simulink model "PV_Mathematical_Model_No_Load"  (R2022a)
settings: Solver=FixedStepAuto  StartTime=0.0  StopTime=5  FixedStep=1e-5  RelTol=1e-3
libraries: simulink x1, spspowerguiLib x1
settings Model: Creator=nikos  LastModifiedBy=nikos

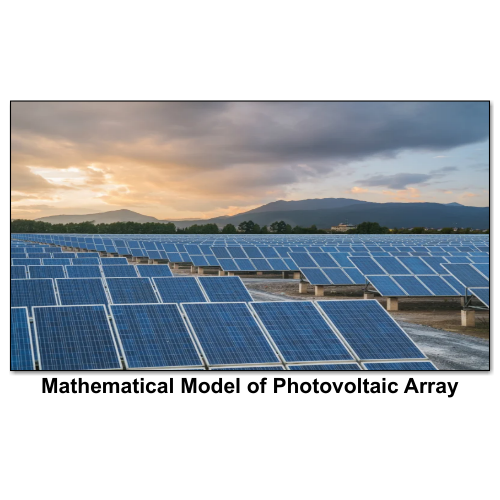
[thumbnail: Simulink's stored preview of the top-level diagram]
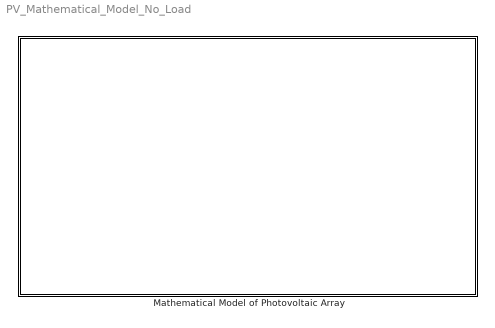
== system PV_Mathematical_Model_No_Load ==
  Mathematical Model of Photovoltaic Array : Subsystem
      mask Display: image('$imagefile'); % Use "Edit Image" on toolstrip to change.

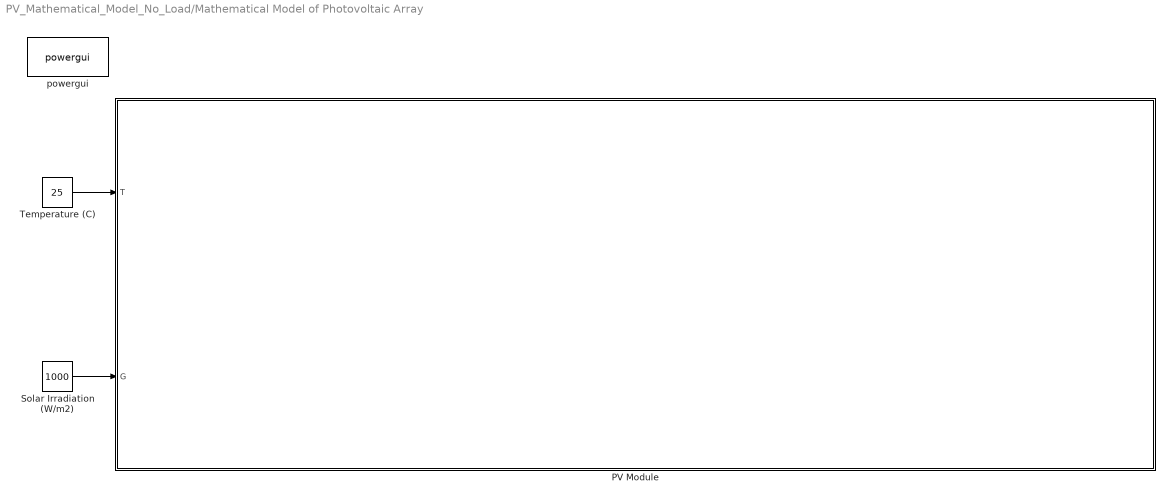
== system PV_Mathematical_Model_No_Load/Mathematical Model of Photovoltaic Array ==
  PV Module : Subsystem
  Solar Irradiation (W/m2) : Constant  Value=1000
  Temperature (C) : Constant  Value=25
  powergui : spspowerguiLib/powergui  Priority=1  SimulationMode=Discrete  SampleTime=50e-6  frequency=60  Iterations=50  frequencyindice=0  Pbase=100e6  ErrMax=1e-4  UnitsV=kV  UnitsW=MW  buscounter=0  FunctionMessages=off  echomessages=off  EnableUseOfTLC=off  CurrentSourceSwitches=off  DisableSnubberDevices=off  DisableRonSwitches=off  DisableVfSwitches=off  DisplayEquations=off  AutomaticDiscreteSolvers=off  SolverType=Tustin/Backward Euler (TBE)  Interpol=off  ExternalGateDelay=off  methode=off  Ts=100  x0status=blocks  SPID=on  SwTol=0  HookPort=off  NonlinearTolerance=1e-4  nMaxIteration=100  ContinueOnMaxIteration=off  RestoreLinks=warning  ResistiveCurrentMeasurement=off  Frange=[0:2:500]  Ylog=off  Xlog=on  ShowGrid=off  save=off  variable=ZData  structure=0  ZoomFFT=off  StartTime=0.0  cycles=1  DisplayStyle=1  fundamental=60  FreqAxis=off  MaxFrequency=1000  frequencyindicesteady=1  RmsSteady=1  display=off
  wires:
  Solar Irradiation (W/m2)/1 -> PV Module/2(G)
  Temperature (C)/1 -> PV Module/1(T)

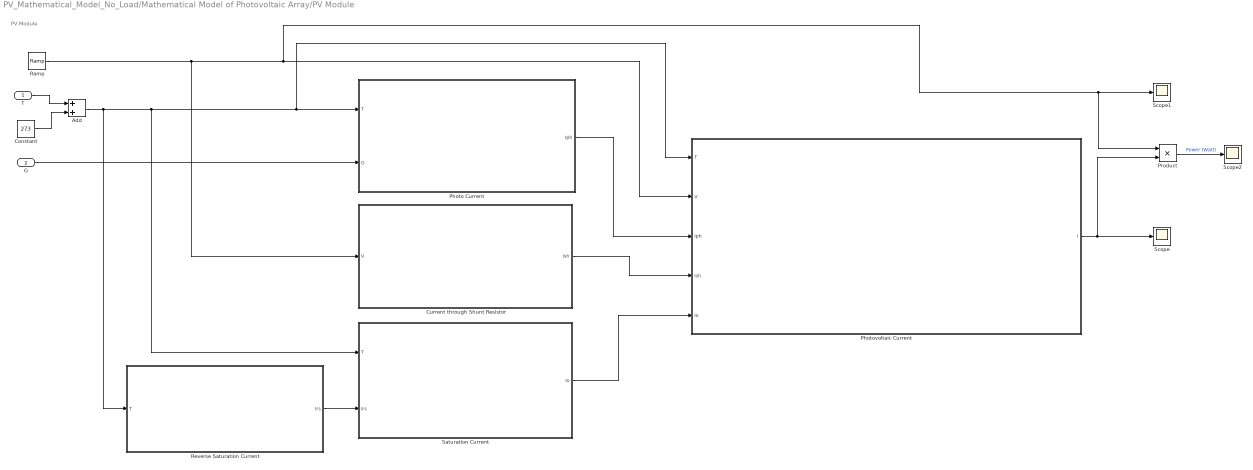
== system PV_Mathematical_Model_No_Load/Mathematical Model of Photovoltaic Array/PV Module ==
  note: PV Module
  T : Inport
  G : Inport  Port=2
  Add : Sum
  Constant : Constant  Value=273
  Current through Shunt Resistor : Subsystem
  Photo Current : Subsystem
  Photovoltaic Current : Subsystem
  Product : Product
  Ramp : simulink/Sources/Ramp  slope=10  start=0  InitialOutput=0
  Reverse Saturation Current : Subsystem
  Saturation Current : Subsystem
  Scope : Scope
  Scope1 : Scope
  Scope2 : Scope
  wires:
  Add/1 -> Reverse Saturation Current/1(T), Photovoltaic Current/1(T), Photo Current/1(T), Saturation Current/1(T)
  Photo Current/1(Iph) -> Photovoltaic Current/3(Iph)
  Current through Shunt Resistor/1(Ish) -> Photovoltaic Current/4(Ish)
  Ramp/1 -> Photovoltaic Current/2(V), Scope1/1, Product/1, Current through Shunt Resistor/1(V)
  G/1 -> Photo Current/2(G)
  T/1 -> Add/1
  Saturation Current/1(Io) -> Photovoltaic Current/5(Io)
  Constant/1 -> Add/2
  Reverse Saturation Current/1(Irs) -> Saturation Current/2(Irs)
  Photovoltaic Current/1(I) -> Scope/1, Product/2
  Product/1 -> Scope2/1  "Power (Watt)"

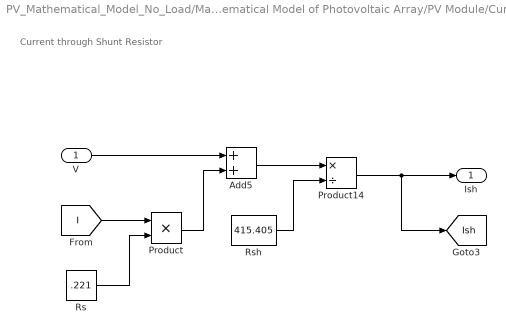
== system PV_Mathematical_Model_No_Load/Mathematical Model of Photovoltaic Array/PV Module/Current through Shunt Resistor ==
  note: Current through Shunt Resistor
  V : Inport
  Add5 : Sum
  Product : Product
  Product14 : Product  Inputs=*/
  Rs : Constant  Value=.221
  Rsh : Constant  Value=415.405
  Ish : Outport
  tag scope: Ish=global
  wires:
  Product14/1 -> Ish/1, [Ish]
  Product/1 -> Add5/2
  Add5/1 -> Product14/1
  [I] -> Product/1
  V/1 -> Add5/1
  Rs/1 -> Product/2
  Rsh/1 -> Product14/2

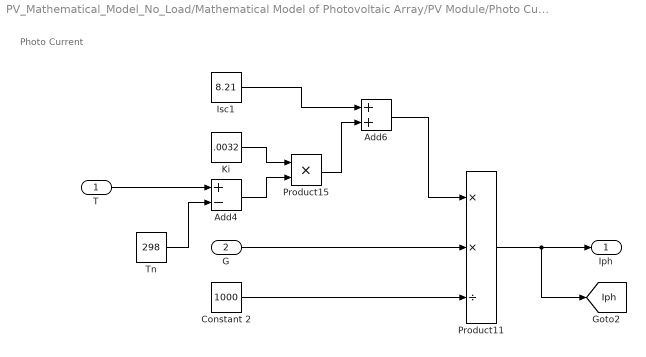
== system PV_Mathematical_Model_No_Load/Mathematical Model of Photovoltaic Array/PV Module/Photo Current ==
  note: Photo Current
  T : Inport
  G : Inport  Port=2
  Add4 : Sum  Inputs=+-
  Add6 : Sum
  Constant 2 : Constant  Value=1000
  Isc1 : Constant  Value=8.21
  Ki : Constant  Value=.0032
  Product11 : Product  Inputs=**/
  Product15 : Product
  Tn : Constant  Value=298
  Iph : Outport
  tag scope: Iph=global
  wires:
  Tn/1 -> Add4/2
  G/1 -> Product11/2
  Add4/1 -> Product15/2
  Ki/1 -> Product15/1
  Product15/1 -> Add6/2
  Add6/1 -> Product11/1
  Product11/1 -> Iph/1, [Iph]
  Isc1/1 -> Add6/1
  Constant 2/1 -> Product11/3
  T/1 -> Add4/1

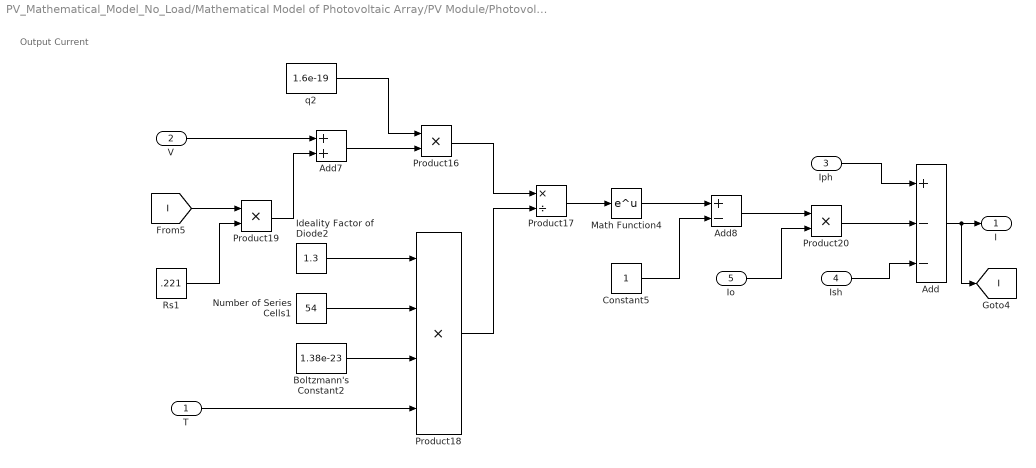
== system PV_Mathematical_Model_No_Load/Mathematical Model of Photovoltaic Array/PV Module/Photovoltaic Current ==
  note: Output Current
  T : Inport
  V : Inport  Port=2
  Iph : Inport  Port=3
  Ish : Inport  Port=4
  Io : Inport  Port=5
  Add : Sum  Inputs=+--
  Add7 : Sum
  Add8 : Sum  Inputs=+-
  Boltzmann's Constant2 : Constant  Value=1.38e-23
  Constant5 : Constant
  Ideality Factor of Diode2 : Constant  Value=1.3
  Math Function4 : Math
  Number of Series Cells1 : Constant  Value=54
  Product16 : Product
  Product17 : Product  Inputs=*/
  Product18 : Product  Inputs=4
  Product19 : Product
  Product20 : Product
  Rs1 : Constant  Value=.221
  q2 : Constant  Value=1.6e-19
  I : Outport
  tag scope: I=global
  wires:
  Ish/1 -> Add/3
  Iph/1 -> Add/1
  Add8/1 -> Product20/1
  Product17/1 -> Math Function4/1
  Product20/1 -> Add/2
  [I] -> Product19/1
  Constant5/1 -> Add8/2
  Math Function4/1 -> Add8/1
  Boltzmann's Constant2/1 -> Product18/3
  q2/1 -> Product16/1
  Product19/1 -> Add7/2
  V/1 -> Add7/1
  Rs1/1 -> Product19/2
  Add7/1 -> Product16/2
  Io/1 -> Product20/2
  T/1 -> Product18/4
  Number of Series Cells1/1 -> Product18/2
  Ideality Factor of Diode2/1 -> Product18/1
  Product18/1 -> Product17/2
  Product16/1 -> Product17/1
  Add/1 -> [I], I/1

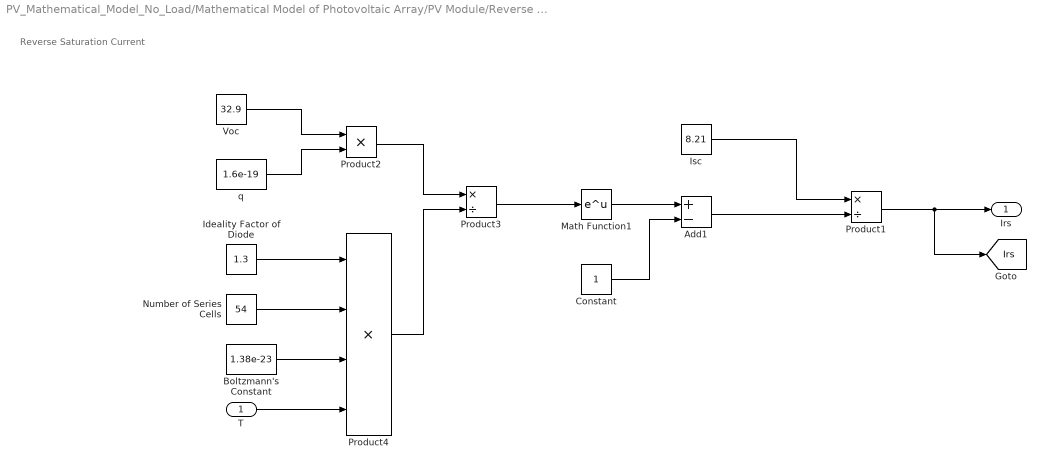
== system PV_Mathematical_Model_No_Load/Mathematical Model of Photovoltaic Array/PV Module/Reverse Saturation Current ==
  note: Reverse Saturation Current
  T : Inport
  Add1 : Sum  Inputs=+-
  Boltzmann's Constant : Constant  Value=1.38e-23
  Constant : Constant
  Ideality Factor of Diode : Constant  Value=1.3
  Isc : Constant  Value=8.21
  Math Function1 : Math
  Number of Series Cells : Constant  Value=54
  Product1 : Product  Inputs=*/
  Product2 : Product
  Product3 : Product  Inputs=*/
  Product4 : Product  Inputs=4
  Voc : Constant  Value=32.9
  q : Constant  Value=1.6e-19
  Irs : Outport
  tag scope: Irs=global
  wires:
  Product1/1 -> Irs/1, [Irs]
  q/1 -> Product2/2
  Number of Series Cells/1 -> Product4/2
  Constant/1 -> Add1/2
  Ideality Factor of Diode/1 -> Product4/1
  Add1/1 -> Product1/2
  T/1 -> Product4/4
  Product4/1 -> Product3/2
  Math Function1/1 -> Add1/1
  Product2/1 -> Product3/1
  Boltzmann's Constant/1 -> Product4/3
  Product3/1 -> Math Function1/1
  Voc/1 -> Product2/1
  Isc/1 -> Product1/1

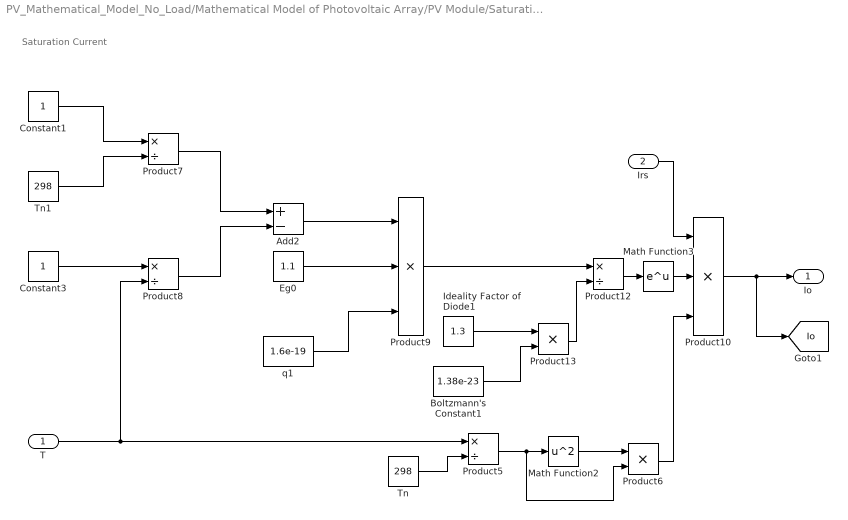
== system PV_Mathematical_Model_No_Load/Mathematical Model of Photovoltaic Array/PV Module/Saturation Current ==
  note: Saturation Current
  T : Inport
  Irs : Inport  Port=2
  Add2 : Sum  Inputs=+-
  Boltzmann's Constant1 : Constant  Value=1.38e-23
  Constant1 : Constant
  Constant3 : Constant
  Eg0 : Constant  Value=1.1
  Ideality Factor of Diode1 : Constant  Value=1.3
  Math Function2 : Math  Operator=square
  Math Function3 : Math
  Product10 : Product  Inputs=3
  Product{5,7..8,12} (4 alike) : Product  Inputs=*/
  Product13 : Product
  Product6 : Product
  Product9 : Product  Inputs=3
  Tn : Constant  Value=298
  Tn1 : Constant  Value=298
  q1 : Constant  Value=1.6e-19
  Io : Outport
  tag scope: Io=global
  wires:
  Irs/1 -> Product10/1
  Ideality Factor of Diode1/1 -> Product13/1
  Product9/1 -> Product12/1
  Product12/1 -> Math Function3/1
  Product8/1 -> Add2/2
  Constant1/1 -> Product7/1
  Boltzmann's Constant1/1 -> Product13/2
  T/1 -> Product8/2, Product5/1
  Math Function2/1 -> Product6/1
  Constant3/1 -> Product8/1
  Product10/1 -> Io/1, [Io]
  Product13/1 -> Product12/2
  Tn1/1 -> Product7/2
  Product6/1 -> Product10/3
  Product5/1 -> Product6/2, Math Function2/1
  Tn/1 -> Product5/2
  Eg0/1 -> Product9/2
  Add2/1 -> Product9/1
  q1/1 -> Product9/3
  Product7/1 -> Add2/1
  Math Function3/1 -> Product10/2
